simulink model "flightControlSystem"  (R2024b)
settings: Solver=ode3  StartTime=0  StopTime=TFinal  FixedStep=Ts  RelTol=1e-3  EnableMultiTasking=on
model workspace (MAT data in the model file):
  CIRCLE_PTS = [19 19 19]
  ZEROS = [0 0 0 0 0 0 0 0 0 0 0 0 ... (1444 elements, 38x38)]
undefined symbols (not defined in the file): codertarget, Controller, DiscIntNeverNeededParam, Discrete, Estimator, g, gray, init, Sensors, Time, Ts, var_acc_angle_N, var_bias_gyr_N, var_gyro_p_N, Vehicle
libraries: simulink x38, slpidlib x4, ctrlSharedLib x4, sharedtransform x3, visiontextngfix x1, parrotlib x1
(part 3 of 3)

== matlab function flightControlSystem/Image Processing System/circle_detection ==
  data: u input; detected output; shape input; way output
function [detected, way] = fcn(u, shape)

persistent landing prev_dist;
if isempty(landing)
    landing = 0;
    prev_dist = inf;  % Initialize previous distance as infinity
end

detected = 0;
way = [0 0 0];
land = 0;

if landing == 1
    way = [0 0 1];
    detected = 1;

else
    [total_pixel, cord_x, cord_y] = detect_circle(u, shape);
    
    if total_pixel >= 1350
        detected = 1;
        center_x = cord_x + 19;
        center_y = cord_y + 19;
    
        % Boundary checks
        if center_x > 120
            center_x = 120;
        end
        if center_y > 160
            center_y = 160;
        end
        
        % Calculate the difference in coordinates and distance
        dif_x = round(60 - center_x);
        dif_y = round(center_y - 80);
        dist = sqrt(dif_x * dif_x + dif_y * dif_y);
    
        % Print the distance as the drone moves
        fprintf('#### CIRCLE - centers: %3.1f %3.1f | dist: %3.1f\n', center_x, center_y, dist);
        
        % Check if the drone is moving away (current distance greater than previous)
        if dist > prev_dist
            fprintf('Drone is moving away, current distance: %3.1f\n', dist);
        end
        
        % Update the previous distance
        prev_dist = dist;

        % Landing condition
        if dist < 15
            land = 1;
            landing = 1;
        end
        
        % Update the movement command
        way_x = dif_x / 130000;
        way_y = dif_y / 130000;
        way = [way_x way_y land];
    end
end

end

function [total_pixel, cord_x, cord_y] = detect_circle(u, shape)

% total_pixel: sum of number of pixels
% cord_x: row coordinate of u
% cord_y: column coordinate of u

[circle_size_x, circle_size_y] = size(shape);
R = 120;  C = 160;

total_pixel = 0;
cord_x = 0;
cord_y = 0;

for i = 1:(R - circle_size_x)
    for j = 1:(C - circle_size_y)
        section = u(i:i+circle_size_x-1, j:j+circle_size_y-1);
        result = sum(~xor(section, shape), 'all');
        if result > total_pixel
            total_pixel = result;
            cord_x = i;
            cord_y = j;
        end
    end
end

end

== matlab function flightControlSystem/Image Processing System/visualize_helper ==
  data: r input; R output; g input; b input; way_x input; way_y input; G output; B output; lx input; ly input; rx input; ry input
function [R,G,B] = fcn(r,g,b, way_x, way_y,  lx,ly, rx,ry)

% completely unnecessary block for algorithm, just for visualize

r(60,80) = 255; g(60,80) = 255; b(60,80) = 255;

if way_x >= 1 && way_y >= 1 && way_x <= 120 && way_y <= 160


% -----------------------------------------------
    x1 = 60; y1 = 80;  x2 = way_x;   y2 = way_y;
    swapepd = 0;
    if abs(y2 - y1) > abs(x2 - x1)
        %disp('[swapped] dy bigger')
        swapepd = 1;
        [x1,y1] = deal(y1,x1);
        [x2,y2] = deal(y2,x2);
        xk = 1; yk = 1;
        if (x2 < x1) xk = -1; end
        if (y2 < y1) yk = -1; end
    else
        xk = -1; yk = -1;
        if (x2 > x1) xk = 1; end
        if (y2 > y1) yk = 1; end

    end
    dy = abs(y2-y1);
    dx = abs(x2-x1);
    % --------------------------------------
    m = 2 * dy;
    slope_error = m - 2*dx;
  
    y = y1;
    for x = x1:xk:x2
        if swapepd == 1
            r(y,x) = 255; g(y,x) = 255; b(y,x) = 255;
        else
            r(x,y) = 255; g(x,y) = 255; b(x,y) = 255;
        end
        
   
        slope_error = slope_error + m;
        if (slope_error > 0)
            y = y + yk;
            slope_error = slope_error - 2 * dx;
        end
    end
end




% --------------------------------------------
x1 = 60; y1 = 80; x2 = lx; y2 = ly;
    swapepd = 0;
    if abs(y2 - y1) > abs(x2 - x1)
        %disp('[swapped] dy bigger')
        swapepd = 1;
        [x1,y1] = deal(y1,x1);
        [x2,y2] = deal(y2,x2);
        xk = 1; yk = 1;
        if (x2 < x1) xk = -1; end
        if (y2 < y1) yk = -1; end
    else
        xk = -1; yk = -1;
        if (x2 > x1) xk = 1; end
        if (y2 > y1) yk = 1; end

    end
    dy = abs(y2-y1);
    dx = abs(x2-x1);
    % --------------------------------------
    m = 2 * dy;
    slope_error = m - 2*dx;
  
    y = y1;
    for x = x1:xk:x2
        if swapepd == 1
            g(y,x) = 255;
        else
            g(x,y) = 255;
        end
        
   
        slope_error = slope_error + m;
        if (slope_error > 0)
            y = y + yk;
            slope_error = slope_error - 2 * dx;
        end
    end
% -----------------------------------------

    x1 = 60; y1 = 80; x2 = rx; y2 = ry;
    swapepd = 0;
    if abs(y2 - y1) >= abs(x2 - x1)
        %disp('[swapped] dy bigger')
        swapepd = 1;
        [x1,y1] = deal(y1,x1);
        [x2,y2] = deal(y2,x2);
        xk = 1; yk = 1;
        if (x2 < x1) xk = -1; end
        if (y2 < y1) yk = -1; end
    else
        xk = -1; yk = -1;
        if (x2 > x1) xk = 1; end
        if (y2 > y1) yk = 1; end

    end
    dy = abs(y2-y1);
    dx = abs(x2-x1);
    % --------------------------------------
    m = 2 * dy;
    slope_error = m - 2*dx;
  
    y = y1;
    for x = x1:xk:x2
        if swapepd == 1
            if x <1 break; end
            g(y,x) = 255;
        else
            g(x,y) = 255;
        end
        
   
        slope_error = slope_error + m;
        if (slope_error > 0)
            y = y + yk;
            slope_error = slope_error - 2 * dx;
        end
    end

b(40:80, 60:90) = 200;
R = r;
G = g;
B = b;
end

== matlab function flightControlSystem/Image Processing System/write_or_not ==
  data: way input; way_out output; in_red input; prev_xy input; way_x output; way_y output
function [way_out, way_x, way_y] = fcn(way, in_red, prev_xy)

x = way(1);
y = way(2);
speed = way(3);

if in_red
    X = x;   Y = y;
    way_x = x;  way_y = y;
else
    X = x;  Y = y; 
    way_x = prev_xy(1);  
    way_y = prev_xy(2);
end

way_out = [X Y speed];

%fprintf('X = %f | Y = %f\n', way_x, way_y);
end

== matlab function flightControlSystem/Control System/Controller/Position Controller/Position error transformation (Earth to Body frame) ==
  data: yaw input; xy_err_earth input; xy_err_body output
function xy_err_body = fcn(yaw,xy_err_earth)

transformation = [cos(yaw), sin(yaw); -sin(yaw),  cos(yaw)];
xy_err_body = transformation * xy_err_earth;


end

== matlab function flightControlSystem/Image Processing System/check_last_way1 ==
  data: u input; is_scan output; in_red output; prev_xy input; DISTANCE input; way output
function [is_scan, in_red, way] = fcn(u, prev_xy, DISTANCE)

% Set the speed factor here (e.g., 0.5 for half speed)
speed_factor = 0.7;

prev_x = prev_xy(1);
prev_y = prev_xy(2);

in_red = u(60, 80);
compare = ~in_red;

is_scan = 0;
way_x = 1;
way_y = 1;
speed = 0;

if prev_x == 0 || prev_y == 0
    is_scan = 1;
else 
    if u(prev_x, prev_y) == 1 

        % endless continue ------------------------------
        [ref_x, ref_y] = middle_point_of_endless_line(u, prev_x, prev_y);

        way_x = prev_x + ref_x;
        way_y = prev_y + ref_y;
        
        if way_y > 160
            if way_x == 120 
                way_x = 120 - mod(way_y, 160);
            elseif way_x == 1 
                way_x = mod(way_y, 160);
            end
            way_y = 160;
            
        elseif way_y < 1
            if way_x == 120 
                way_x = 120 - abs(way_y);
            elseif way_x == 1 
                way_x = abs(way_y); 
            end
            way_y = 1;
            
        elseif way_x < 1
            if way_y == 160
                way_y = 160 - abs(way_x);
            elseif way_y == 1
                way_y = abs(way_x);
            end
            way_x = 1;
            
        elseif way_x > 120
            if way_y == 160
                way_y = 160 - (way_x - 120);
            elseif way_y == 1
                way_y = way_x - 120;
            end
            way_x = 120;
        end

        % Apply speed factor
        speed = 100 * speed_factor;

    else 
        
        % endless disappeared ----------------------------
        if in_red
            distance = line_drawer(60, 80, prev_x, prev_y, u, compare);
            if distance < DISTANCE
                is_scan = 1;
                speed = 0;
            else
                speed = distance * speed_factor;
            end
            
            way_x = prev_x;
            way_y = prev_y;
        else
            is_scan = 1;
            way_x = prev_x;
            way_y = prev_y;
            speed = 40 * speed_factor;
        end

    end
end
way = [way_x, way_y, speed];

end % func end



function [ref_x, ref_y] = middle_point_of_endless_line(u, way_x, way_y)

w = edge_number(way_x, way_y);

if w == 1 || w == 3

    % to right
    iter_y = way_y;
    iter_x = way_x;
    plus_or_minus = 1;
    x_or_y = 0; % 0:y   1:x
    distance = 0;

    while u(iter_x, iter_y) == 1
        if x_or_y == 0
            iter_y = iter_y + plus_or_minus;
        else
            iter_x = iter_x + plus_or_minus;
        end
        distance = distance + 1;
        
        if iter_y > 160
            iter_y = 160;
            x_or_y = 1;
            if iter_x == 120
                plus_or_minus = -1;
            elseif iter_x == 1
                plus_or_minus = 1;
            end
        end
        if iter_x < 1
            break;
        elseif iter_x > 120
            break;
        end
    end
    right = distance;

    % to left
    iter_y = way_y;
    iter_x = way_x;
    plus_or_minus = -1;
    x_or_y = 0; % 0:y   1:x
    distance = 0;
    
    while u(iter_x, iter_y) == 1
        if x_or_y == 0
            iter_y = iter_y + plus_or_minus;
        else
            iter_x = iter_x + plus_or_minus;
        end
        distance = distance + 1;

        if iter_y < 1
            iter_y = 1;
            x_or_y = 1;
            if iter_x == 120
                plus_or_minus = -1;
            elseif iter_x == 1
                plus_or_minus = 1;
            end
        end
        if iter_x < 1
            break
        elseif iter_x > 120
            break
        end
    end
    left = distance;
    
    ref_x = 0;
    diff = right - left;
    
    if abs(diff) >= 7 && abs(diff) < 25
        ref_y = round(diff/2);
    else
        ref_y = 0;
    end

else % ------------------------- 2 & 4 --------------------------
    % to up
    iter_x = way_x;
    iter_y = way_y;
    plus_or_minus = -1;
    x_or_y = 1; % 0:y   1:x
    distance = 0;
    while u(iter_x, iter_y) == 1
        if x_or_y == 0
            iter_y = iter_y + plus_or_minus;
        else
            iter_x = iter_x + plus_or_minus;
        end
        distance = distance + 1;

        if iter_x < 1
            iter_x = 1;
            x_or_y = 0;
            if iter_y == 1
                plus_or_minus = 1;
            elseif iter_y == 160
                plus_or_minus = -1;
            end
        end
        if iter_y > 160
            break
        elseif iter_y < 1
            break
        end
    end
    up = distance;

    % to down
    iter_x = way_x;
    iter_y = way_y;
    plus_or_minus = 1;
    x_or_y = 1; % 0:y   1:x
    distance = 0;
    while u(iter_x, iter_y) == 1
        if x_or_y == 0
            iter_y = iter_y + plus_or_minus;
        else
            iter_x = iter_x + plus_or_minus;
        end
        distance = distance + 1;
        if iter_x > 120
            x_or_y = 0;
            iter_x = 120;
            if iter_y == 1
                plus_or_minus = 1;
            elseif iter_y == 160
                plus_or_minus = -1;
            end
        end
        if iter_y > 160
            break;
        elseif iter_y < 1
            break;
        end
    end
    down = distance;

    diff = down - up;

    ref_y = 0;
    if abs(diff) >= 7 && abs(diff) < 25
        ref_x = round(diff/2);
    else
        ref_x = 0;
    end
end

end

== matlab function flightControlSystem/Image Processing System/speed_calculator ==
  data: way input; X output; Y output
function [X,Y] = fcn(way)

x = way(1);
y = way(2);
speed = way(3);

if speed == 100
    speed = 200;
elseif speed < 60
    speed = 60;
end


X = (60-x) / 10000000 * speed;
Y = (y-80) / 10000000 * speed;


%fprintf(' --- speed: %f | ', speed); fprintf('vectors: X=%.5f | Y=%.5f\n', X, Y);

end

== matlab function flightControlSystem/Control System/Controller/MATLAB Function ==
  data: xy output; x input; z output; y input; z input; t input; zhold input; thold input
function [xy, z] = fcn(x, y, z, t,zhold,thold)
    % Define persistent variables to track the condition state and hold timing
    persistent condition_met hold_start_time last_xy;
    
    % Initialize persistent variables on the first run
    if isempty(condition_met)
        condition_met = 0;             % Initialize as 0 (no conditions met)
        hold_start_time = -1;          % Initial hold start time (inactive)
        last_xy = [x; y];              % Initialize last known x and y position as [2 x 1]
    end
    
    % Calculate the distance from the origin
    dist = sqrt(x^2 + y^2);
    
    % Define thresholds
    threshold1 = 1.6778;  % First threshold for z = -0.5
    threshold2 = 4.099;   % Second threshold for z = 0
    
    % Check conditions
    if condition_met == 0 && dist > threshold1
        z = single(-zhold);             % Set z to -0.5 when the first threshold is crossed
        condition_met = 1;            % Update condition_met to 1
        hold_start_time = t;          % Set hold start time to the current time
        last_xy = [x; y];             % Save the current x and y position
    elseif condition_met == 1
        if t - hold_start_time < thold    % Check if 3 seconds have passed
            z = single(-zhold);         % Hold z at -0.5
            xy = last_xy;             % Keep x, y at the saved position
            return                     % Exit to hold position without updating x, y
        else
            z = single(-1);           % After 3 seconds, set z back to -1
            condition_met = 1.5;      % Set intermediate state to resume movement
        end
    elseif condition_met == 1.5 && dist > threshold2
        z = single(0);                % Set z to 0 when the second threshold is crossed
        condition_met = 2;            % Update condition_met to 2
    elseif condition_met == 2
        z = single(0);                % Keep z at 0 after the second condition is met
    end
    
    % If conditions are met for x, y to move, update x, y normally
    xy = [x; y];                      % Ensure xy output is consistently [2 x 1] format
end

== matlab function flightControlSystem/Image Processing System/opposite_way ==
  data: way_x output; prev_xy input; way_y output
function [way_x, way_y] = fcn(prev_xy)

    x = prev_xy(1);
    y = prev_xy(2);
    
    if x == 0 || y == 0
        way_x = 0;
        way_y = 0;
    else
        way_x = 60 + (60 - x) + 1;
        way_y = 80 + (80 - y) + 1;
    end

    %fprintf('opposite: %.0f %.0f -> %.0f %.0f\n', x, y, way_x, way_y);
end

== matlab function flightControlSystem/Image Processing System/center_vector_x ==
  data: u input; slide_x output
function slide_x = fcn(u)
c1 = 60; 
c2 = 80;
left_p = 0;
right_p = 0;
middle_point = u(c1, c2);
compare = ~middle_point;
for i = c2:-1:60 % <---  look left
    if u(c1, i) == compare
        left_p = i;
        break
    end
end
for i = c2:100 % --->   look right
    if u(c1, i) == compare
        right_p = i;
        break
    end
end

slide_x = 0;
if left_p ~= 0 && right_p ~= 0 % in line
    if middle_point == 1
        vr = right_p - c2;  % length right 
        vl = c2 - left_p;   % length left
        diff = vr-vl;
        slide_x = get_speed(diff) * 20;
    end
end
end

function T = get_speed(t)

if t > 0
    if t < 1
        T = 0.000001;
    elseif t < 5
        T = 0.000002;
    elseif t < 10
        T = 0.000003;
    elseif t < 15
        T = 0.000004;
    elseif t < 20
        T = 0.000005;
    else
        T = 0.000006;
    end
else
    if t < -20
        T = -0.000006;
    elseif t < -15
        T = -0.000005;
    elseif t < -10
        T = -0.000004;
    elseif t < -5
        T = -0.000003;
    elseif t < -1
        T = -0.000002;
    else
        T = -0.000001;
    end
end

end

== matlab function flightControlSystem/Image Processing System/range_points ==
  data: x input; x1 output; y input; ref input; y1 output; x2 output; y2 output
function [x1,y1, x2,y2] = get_range_points(x,y, ref)

% x1, y1 are left
% x2, y2 are right 
% according to center-to-edge vector.

W = edge_number(x,y);

if W == 1
    y1 = y - ref;
    if y1 < 1
        x1 = x - y1;
        y1 = 1;
    else
        x1 = x;
    end

    y2 = y + ref;
    if y2 > 160
        x2 = y2-160;
        y2 = 160;
    else
        x2 = x;
    end
elseif W == 2
    x1 = x + ref;
    if x1 > 120
        y1 = x1 - 120;
        x1 = 120;
    else
        y1 = y;
    end

    x2 = x - ref;
    if x2 < 1
        y2 = abs(x2) + 1;
        x2 = 1;
    else
        y2 = y;
    end
elseif W == 4
    x1 = x - ref;
    if x1 < 1
        y1 = 160 + x1;
        x1 = 1;
    else
        y1 = 160;
    end

    x2 = x + ref;
    if x2 > 120
        y2 = 160 - (x2 - 120);
        x2 = 120;
    else
        y2 = y;
    end
elseif W == 3
    y1 = y + ref;
    if y1 > 160
        x1 = 120 - (y1-160);
        y1 = 160;
    else
        x1 = x;
    end

    y2 = y - ref;
    if y2 < 1
        x2 = 120 + y2;
        y2 = 1;
    else
        x2 = x;
    end
else
    x1 = 1; y1 = 1;
    x2 = 1; y2 = 2;
end

%fprintf('range_points: %.0f-%.0f  to  %.0f-%.0f\n', x1,y1, x2,y2);

end

== stateflow chart flightControlSystem/Control System/Path Planning/Chart ==
  state hover
    xout = 0;
    yout = 0;
    zout = -1.1;
  state go
    xout = xout + xin;
    yout = yout + yin;
    zout = -1.1;
  state land
    zout = zout + 0.004;
    xout = xout;
    yout = yout;
  (default) -> hover
  go -> land : [land == 1]
  hover -> go : [after(2, sec)]
  data: xout output; yout output; zout output; yin input; xin input; land input
